simulink model "CommunicationControl"  (R2023a)
settings: Solver=VariableStepAuto  StartTime=0.0  StopTime=10.0  RelTol=1e-3
settings Model: Creator=aan18022  LastModifiedBy=aan18022

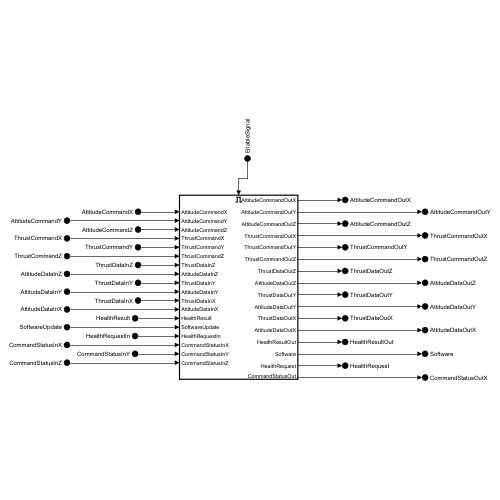
[thumbnail: Simulink's stored preview of the top-level diagram]
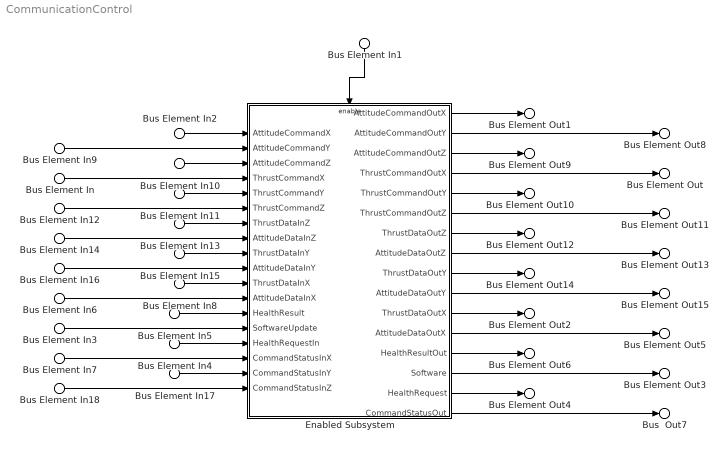
== system CommunicationControl ==
  Bus Element In1 : Inport  PortName=EnableSignal
  Bus Element In2 : Inport  Port=2  PortName=AttitudeCommandX
  Bus Element In3 : Inport  Port=3  PortName=SoftwareUpdate
  Bus Element In4 : Inport  Port=4  PortName=HealthRequestIn
  Bus Element In5 : Inport  Port=5  PortName=HealthResult
  Bus Element In6 : Inport  Port=6  PortName=AttitudeDataInX
  Bus Element In7 : Inport  Port=7  PortName=CommandStatusInX
  Bus Element In : Inport  Port=8  PortName=ThrustCommandX
  Bus Element In8 : Inport  Port=9  PortName=ThrustDataInX
  Bus Element In9 : Inport  Port=10  PortName=AttitudeCommandY
  Bus Element In10 : Inport  Port=11  PortName=AttitudeCommandZ
  Bus Element In11 : Inport  Port=12  PortName=ThrustCommandY
  Bus Element In12 : Inport  Port=13  PortName=ThrustCommandZ
  Bus Element In13 : Inport  Port=14  PortName=ThrustDataInZ
  Bus Element In14 : Inport  Port=15  PortName=AttitudeDataInZ
  Bus Element In15 : Inport  Port=16  PortName=ThrustDataInY
  Bus Element In16 : Inport  Port=17  PortName=AttitudeDataInY
  Bus Element In17 : Inport  Port=18  PortName=CommandStatusInY
  Bus Element In18 : Inport  Port=19  PortName=CommandStatusInZ
  Enabled Subsystem : Subsystem  TreatAsAtomicUnit=on
  Bus Element Out3 : Outport  PortName=Software
  Bus Element Out4 : Outport  Port=2  PortName=HealthRequest
  Bus Element Out5 : Outport  Port=3  PortName=AttitudeDataOutX
  Bus Element Out6 : Outport  Port=4  PortName=HealthResultOut
  Bus Element Out1 : Outport  Port=5  PortName=AttitudeCommandOutX
  Bus  Out7 : Outport  Port=6  PortName=CommandStatusOutX
  Bus Element Out : Outport  Port=7  VectorParamsAs1DForOutWhenUnconnected=off  PortName=ThrustCommandOutX
  Bus Element Out2 : Outport  Port=8  PortName=ThrustDataOutX
  Bus Element Out8 : Outport  Port=9  PortName=AttitudeCommandOutY
  Bus Element Out9 : Outport  Port=10  PortName=AttitudeCommandOutZ
  Bus Element Out10 : Outport  Port=11  PortName=ThrustCommandOutY
  Bus Element Out11 : Outport  Port=12  PortName=ThrustCommandOutZ
  Bus Element Out12 : Outport  Port=13  PortName=ThrustDataOutZ
  Bus Element Out13 : Outport  Port=14  PortName=AttitudeDataOutZ
  Bus Element Out14 : Outport  Port=15  PortName=ThrustDataOutY
  Bus Element Out15 : Outport  Port=16  PortName=AttitudeDataOutY
  wires:
  Bus Element In1/1 -> Enabled Subsystem/Enable
  Bus Element In2/1 -> Enabled Subsystem/1(AttitudeCommandX)
  Bus Element In3/1 -> Enabled Subsystem/14(SoftwareUpdate)
  Bus Element In4/1 -> Enabled Subsystem/15(HealthRequestIn)
  Bus Element In5/1 -> Enabled Subsystem/13(HealthResult)
  Bus Element In6/1 -> Enabled Subsystem/12(AttitudeDataInX)
  Bus Element In7/1 -> Enabled Subsystem/16(CommandStatusInX)
  Enabled Subsystem/14(Software) -> Bus Element Out3/1
  Enabled Subsystem/15(HealthRequest) -> Bus Element Out4/1
  Enabled Subsystem/12(AttitudeDataOutX) -> Bus Element Out5/1
  Enabled Subsystem/13(HealthResultOut) -> Bus Element Out6/1
  Enabled Subsystem/1(AttitudeCommandOutX) -> Bus Element Out1/1
  Enabled Subsystem/16(CommandStatusOut) -> Bus  Out7/1
  Bus Element In/1 -> Enabled Subsystem/4(ThrustCommandX)
  Enabled Subsystem/4(ThrustCommandOutX) -> Bus Element Out/1
  Bus Element In8/1 -> Enabled Subsystem/11(ThrustDataInX)
  Enabled Subsystem/11(ThrustDataOutX) -> Bus Element Out2/1
  Enabled Subsystem/2(AttitudeCommandOutY) -> Bus Element Out8/1
  Enabled Subsystem/3(AttitudeCommandOutZ) -> Bus Element Out9/1
  Enabled Subsystem/5(ThrustCommandOutY) -> Bus Element Out10/1
  Enabled Subsystem/6(ThrustCommandOutZ) -> Bus Element Out11/1
  Enabled Subsystem/7(ThrustDataOutZ) -> Bus Element Out12/1
  Enabled Subsystem/8(AttitudeDataOutZ) -> Bus Element Out13/1
  Enabled Subsystem/9(ThrustDataOutY) -> Bus Element Out14/1
  Enabled Subsystem/10(AttitudeDataOutY) -> Bus Element Out15/1
  Bus Element In9/1 -> Enabled Subsystem/2(AttitudeCommandY)
  Bus Element In10/1 -> Enabled Subsystem/3(AttitudeCommandZ)
  Bus Element In11/1 -> Enabled Subsystem/5(ThrustCommandY)
  Bus Element In12/1 -> Enabled Subsystem/6(ThrustCommandZ)
  Bus Element In13/1 -> Enabled Subsystem/7(ThrustDataInZ)
  Bus Element In14/1 -> Enabled Subsystem/8(AttitudeDataInZ)
  Bus Element In15/1 -> Enabled Subsystem/9(ThrustDataInY)
  Bus Element In16/1 -> Enabled Subsystem/10(AttitudeDataInY)
  Bus Element In17/1 -> Enabled Subsystem/17(CommandStatusInY)
  Bus Element In18/1 -> Enabled Subsystem/18(CommandStatusInZ)

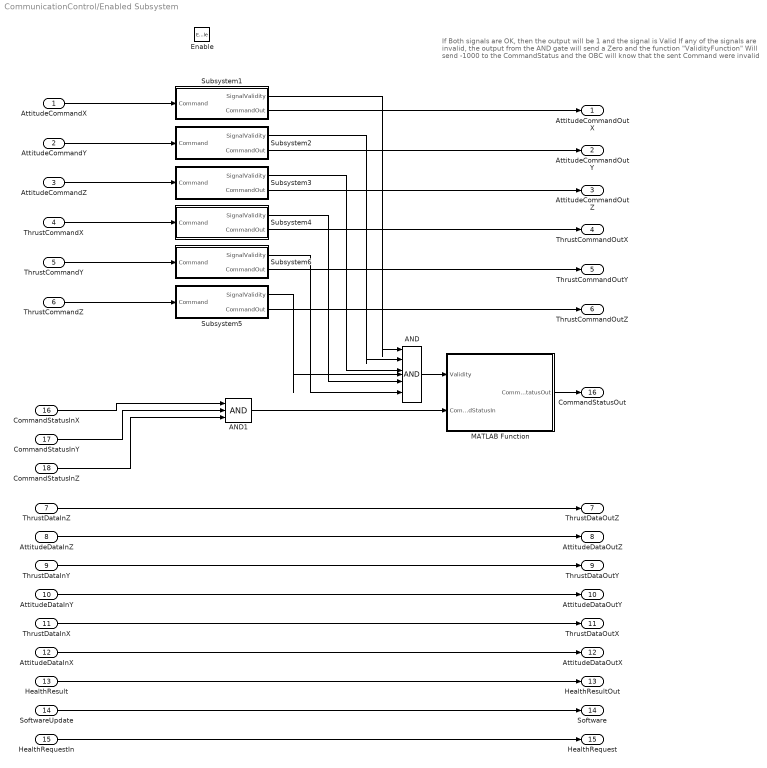
== system CommunicationControl/Enabled Subsystem ==
  note: If Both signals are OK, then the output will be 1 and the signal is Valid
      |
      | If any of the signals are invalid, the output from the AND gate will send a Zero and the function "ValidityFunction" Will send -1000 to the  CommandStatus and the OBC will know that the sent Command were invalid
  AttitudeCommandX : Inport
  AttitudeCommandY : Inport  Port=2
  AttitudeCommandZ : Inport  Port=3
  ThrustCommandX : Inport  Port=4
  ThrustCommandY : Inport  Port=5
  ThrustCommandZ : Inport  Port=6
  ThrustDataInZ : Inport  Port=7
  AttitudeDataInZ : Inport  Port=8
  ThrustDataInY : Inport  Port=9
  AttitudeDataInY : Inport  Port=10
  ThrustDataInX : Inport  Port=11
  AttitudeDataInX : Inport  Port=12
  HealthResult : Inport  Port=13
  SoftwareUpdate : Inport  Port=14
  HealthRequestIn : Inport  Port=15
  CommandStatusInX : Inport  Port=16
  CommandStatusInY : Inport  Port=17
  CommandStatusInZ : Inport  Port=18
  Enable : EnablePort
  AND : Logic  Inputs=6  IconShape=distinctive  AllPortsSameDT=off  OutDataTypeStr=boolean
  AND1 : Logic  Inputs=3  IconShape=distinctive  AllPortsSameDT=off  OutDataTypeStr=boolean
  MATLAB Function : MATLAB Function  TreatAsAtomicUnit=on
  Subsystem1 : Subsystem
  Subsystem2 : Subsystem
  Subsystem3 : Subsystem
  Subsystem4 : Subsystem
  Subsystem5 : Subsystem
  Subsystem6 : Subsystem
  AttitudeCommandOutX : Outport
  AttitudeCommandOutY : Outport  Port=2
  AttitudeCommandOutZ : Outport  Port=3
  ThrustCommandOutX : Outport  Port=4
  ThrustCommandOutY : Outport  Port=5
  ThrustCommandOutZ : Outport  Port=6
  ThrustDataOutZ : Outport  Port=7
  AttitudeDataOutZ : Outport  Port=8
  ThrustDataOutY : Outport  Port=9
  AttitudeDataOutY : Outport  Port=10
  ThrustDataOutX : Outport  Port=11
  AttitudeDataOutX : Outport  Port=12
  HealthResultOut : Outport  Port=13
  Software : Outport  Port=14
  HealthRequest : Outport  Port=15
  CommandStatusOut : Outport  Port=16
  wires:
  Subsystem1/2(CommandOut) -> AttitudeCommandOutX/1
  SoftwareUpdate/1 -> Software/1
  AttitudeDataInX/1 -> AttitudeDataOutX/1
  HealthResult/1 -> HealthResultOut/1
  HealthRequestIn/1 -> HealthRequest/1
  AND/1 -> MATLAB Function/1(Validity)
  MATLAB Function/1(CommandStatusOut) -> CommandStatusOut/1
  ThrustDataInX/1 -> ThrustDataOutX/1
  ThrustCommandX/1 -> Subsystem4/1(Command)
  Subsystem4/2(CommandOut) -> ThrustCommandOutX/1
  AttitudeCommandX/1 -> Subsystem1/1(Command)
  AttitudeCommandZ/1 -> Subsystem3/1(Command)
  AttitudeCommandY/1 -> Subsystem2/1(Command)
  ThrustCommandY/1 -> Subsystem6/1(Command)
  ThrustCommandZ/1 -> Subsystem5/1(Command)
  Subsystem1/1(SignalValidity) -> AND/1
  Subsystem2/1(SignalValidity) -> AND/2
  Subsystem3/1(SignalValidity) -> AND/3
  Subsystem4/1(SignalValidity) -> AND/4
  Subsystem6/1(SignalValidity) -> AND/5
  Subsystem5/1(SignalValidity) -> AND/6
  Subsystem2/2(CommandOut) -> AttitudeCommandOutY/1
  Subsystem3/2(CommandOut) -> AttitudeCommandOutZ/1
  Subsystem6/2(CommandOut) -> ThrustCommandOutY/1
  Subsystem5/2(CommandOut) -> ThrustCommandOutZ/1
  AttitudeDataInY/1 -> AttitudeDataOutY/1
  AttitudeDataInZ/1 -> AttitudeDataOutZ/1
  ThrustDataInZ/1 -> ThrustDataOutZ/1
  ThrustDataInY/1 -> ThrustDataOutY/1
  AND1/1 -> MATLAB Function/2(CommandStatusIn)
  CommandStatusInX/1 -> AND1/1
  CommandStatusInY/1 -> AND1/2
  CommandStatusInZ/1 -> AND1/3

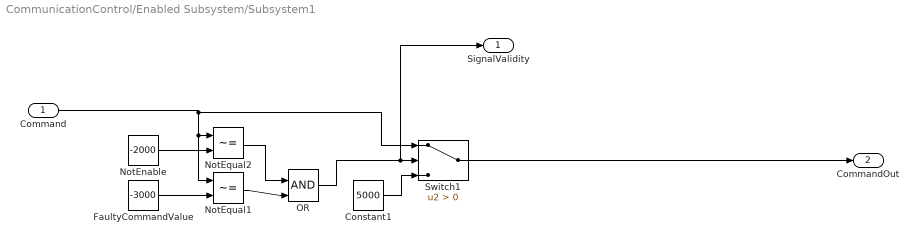
== system CommunicationControl/Enabled Subsystem/Subsystem1 ==
  Command : Inport
  Constant1 : Constant  Value=5000
  FaultyCommandValue : Constant  Value=-3000
  NotEnable : Constant  Value=-2000
  NotEqual1 : RelationalOperator  Operator=~=  OutDataTypeStr=boolean  RndMeth=Simplest  InputSameDT=off
  NotEqual2 : RelationalOperator  Operator=~=  OutDataTypeStr=boolean  RndMeth=Simplest  InputSameDT=off
  OR : Logic  IconShape=distinctive  AllPortsSameDT=off  OutDataTypeStr=boolean
  Switch1 : Switch  Criteria=u2 > Threshold  SaturateOnIntegerOverflow=off  InputSameDT=off
  SignalValidity : Outport
  CommandOut : Outport  Port=2
  wires:
  FaultyCommandValue/1 -> NotEqual1/2
  Switch1/1 -> CommandOut/1
  Constant1/1 -> Switch1/3
  Command/1 -> NotEqual2/1, NotEqual1/1, Switch1/1
  NotEqual1/1 -> OR/2
  NotEnable/1 -> NotEqual2/2
  NotEqual2/1 -> OR/1
  OR/1 -> SignalValidity/1, Switch1/2

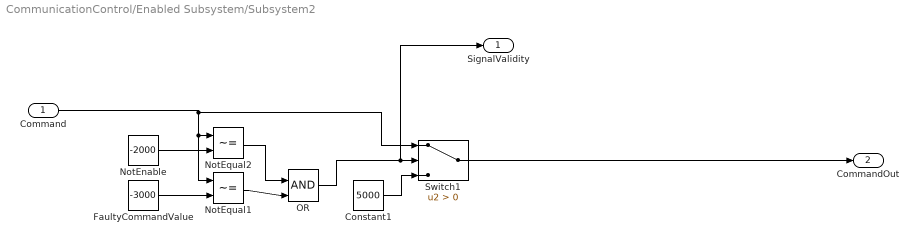
== system CommunicationControl/Enabled Subsystem/Subsystem2 ==
  Command : Inport
  Constant1 : Constant  Value=5000
  FaultyCommandValue : Constant  Value=-3000
  NotEnable : Constant  Value=-2000
  NotEqual1 : RelationalOperator  Operator=~=  OutDataTypeStr=boolean  RndMeth=Simplest  InputSameDT=off
  NotEqual2 : RelationalOperator  Operator=~=  OutDataTypeStr=boolean  RndMeth=Simplest  InputSameDT=off
  OR : Logic  IconShape=distinctive  AllPortsSameDT=off  OutDataTypeStr=boolean
  Switch1 : Switch  Criteria=u2 > Threshold  SaturateOnIntegerOverflow=off  InputSameDT=off
  SignalValidity : Outport
  CommandOut : Outport  Port=2
  wires:
  FaultyCommandValue/1 -> NotEqual1/2
  Switch1/1 -> CommandOut/1
  Constant1/1 -> Switch1/3
  Command/1 -> NotEqual2/1, NotEqual1/1, Switch1/1
  NotEqual1/1 -> OR/2
  NotEnable/1 -> NotEqual2/2
  NotEqual2/1 -> OR/1
  OR/1 -> SignalValidity/1, Switch1/2

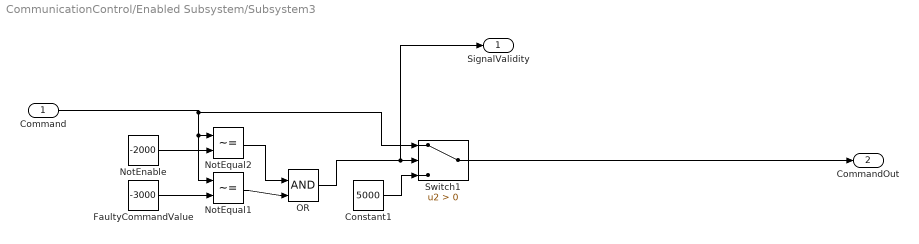
== system CommunicationControl/Enabled Subsystem/Subsystem3 ==
  Command : Inport
  Constant1 : Constant  Value=5000
  FaultyCommandValue : Constant  Value=-3000
  NotEnable : Constant  Value=-2000
  NotEqual1 : RelationalOperator  Operator=~=  OutDataTypeStr=boolean  RndMeth=Simplest  InputSameDT=off
  NotEqual2 : RelationalOperator  Operator=~=  OutDataTypeStr=boolean  RndMeth=Simplest  InputSameDT=off
  OR : Logic  IconShape=distinctive  AllPortsSameDT=off  OutDataTypeStr=boolean
  Switch1 : Switch  Criteria=u2 > Threshold  SaturateOnIntegerOverflow=off  InputSameDT=off
  SignalValidity : Outport
  CommandOut : Outport  Port=2
  wires:
  FaultyCommandValue/1 -> NotEqual1/2
  Switch1/1 -> CommandOut/1
  Constant1/1 -> Switch1/3
  Command/1 -> NotEqual2/1, NotEqual1/1, Switch1/1
  NotEqual1/1 -> OR/2
  NotEnable/1 -> NotEqual2/2
  NotEqual2/1 -> OR/1
  OR/1 -> SignalValidity/1, Switch1/2

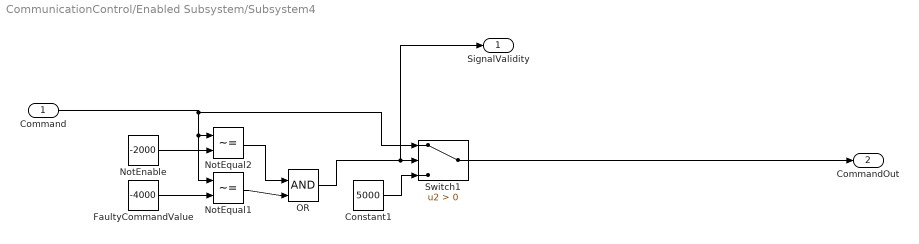
== system CommunicationControl/Enabled Subsystem/Subsystem4 ==
  Command : Inport
  Constant1 : Constant  Value=5000
  FaultyCommandValue : Constant  Value=-4000
  NotEnable : Constant  Value=-2000
  NotEqual1 : RelationalOperator  Operator=~=  OutDataTypeStr=boolean  RndMeth=Simplest  InputSameDT=off
  NotEqual2 : RelationalOperator  Operator=~=  OutDataTypeStr=boolean  RndMeth=Simplest  InputSameDT=off
  OR : Logic  IconShape=distinctive  AllPortsSameDT=off  OutDataTypeStr=boolean
  Switch1 : Switch  Criteria=u2 > Threshold  SaturateOnIntegerOverflow=off  InputSameDT=off
  SignalValidity : Outport
  CommandOut : Outport  Port=2
  wires:
  FaultyCommandValue/1 -> NotEqual1/2
  Switch1/1 -> CommandOut/1
  Constant1/1 -> Switch1/3
  Command/1 -> NotEqual2/1, NotEqual1/1, Switch1/1
  NotEqual1/1 -> OR/2
  NotEnable/1 -> NotEqual2/2
  NotEqual2/1 -> OR/1
  OR/1 -> SignalValidity/1, Switch1/2

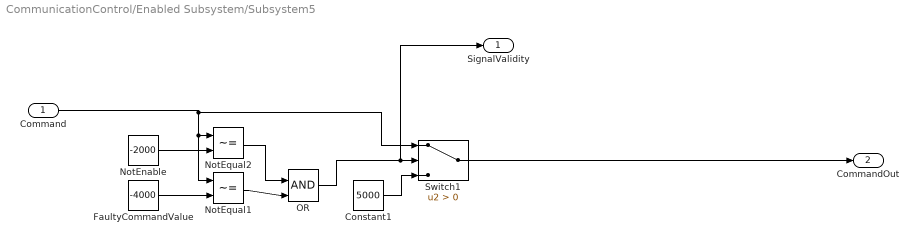
== system CommunicationControl/Enabled Subsystem/Subsystem5 ==
  Command : Inport
  Constant1 : Constant  Value=5000
  FaultyCommandValue : Constant  Value=-4000
  NotEnable : Constant  Value=-2000
  NotEqual1 : RelationalOperator  Operator=~=  OutDataTypeStr=boolean  RndMeth=Simplest  InputSameDT=off
  NotEqual2 : RelationalOperator  Operator=~=  OutDataTypeStr=boolean  RndMeth=Simplest  InputSameDT=off
  OR : Logic  IconShape=distinctive  AllPortsSameDT=off  OutDataTypeStr=boolean
  Switch1 : Switch  Criteria=u2 > Threshold  SaturateOnIntegerOverflow=off  InputSameDT=off
  SignalValidity : Outport
  CommandOut : Outport  Port=2
  wires:
  FaultyCommandValue/1 -> NotEqual1/2
  Switch1/1 -> CommandOut/1
  Constant1/1 -> Switch1/3
  Command/1 -> NotEqual2/1, NotEqual1/1, Switch1/1
  NotEqual1/1 -> OR/2
  NotEnable/1 -> NotEqual2/2
  NotEqual2/1 -> OR/1
  OR/1 -> SignalValidity/1, Switch1/2

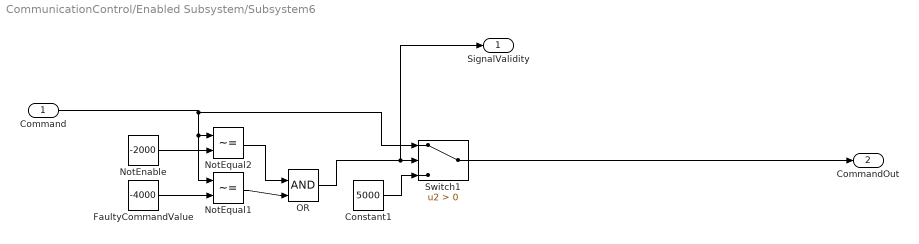
== system CommunicationControl/Enabled Subsystem/Subsystem6 ==
  Command : Inport
  Constant1 : Constant  Value=5000
  FaultyCommandValue : Constant  Value=-4000
  NotEnable : Constant  Value=-2000
  NotEqual1 : RelationalOperator  Operator=~=  OutDataTypeStr=boolean  RndMeth=Simplest  InputSameDT=off
  NotEqual2 : RelationalOperator  Operator=~=  OutDataTypeStr=boolean  RndMeth=Simplest  InputSameDT=off
  OR : Logic  IconShape=distinctive  AllPortsSameDT=off  OutDataTypeStr=boolean
  Switch1 : Switch  Criteria=u2 > Threshold  SaturateOnIntegerOverflow=off  InputSameDT=off
  SignalValidity : Outport
  CommandOut : Outport  Port=2
  wires:
  FaultyCommandValue/1 -> NotEqual1/2
  Switch1/1 -> CommandOut/1
  Constant1/1 -> Switch1/3
  Command/1 -> NotEqual2/1, NotEqual1/1, Switch1/1
  NotEqual1/1 -> OR/2
  NotEnable/1 -> NotEqual2/2
  NotEqual2/1 -> OR/1
  OR/1 -> SignalValidity/1, Switch1/2

== matlab function CommunicationControl/Enabled Subsystem/MATLAB Function ==
  data: Validity input; Out output; CommandStatusIn input
function Out = fcn(Validity, CommandStatusIn)

if Validity ==1
    Out = CommandStatusIn;
else
    Out = -1000;
end
